simulink model "lab2_1"  (R2023b)
settings: Solver=VariableStepAuto  StartTime=0.0  StopTime=20.0  MaxStep=0.001  RelTol=1e-3
settings Model: Creator=insomnia  LastModifiedBy=insomnia

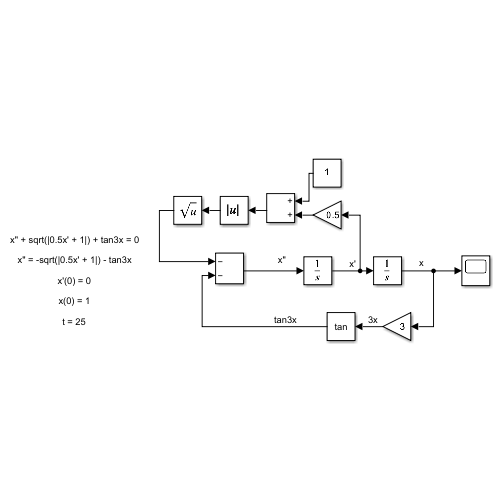
[thumbnail: Simulink's stored preview of the top-level diagram]
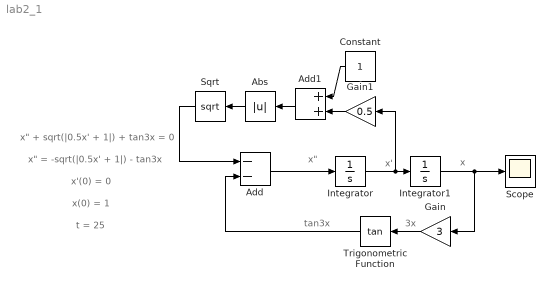
== system lab2_1 ==
  note: 3x
  note: tan3x
  note: x" + sqrt(|0.5x' + 1|) + tan3x = 0
  note: x" = -sqrt(|0.5x' + 1|) - tan3x
  note: x'
  note: x"
  note: x
  note: x'(0) = 0
  note: x(0) = 1
  note: t = 25
  Abs : Abs  SaturateOnIntegerOverflow=off
  Add : Sum  Inputs=--
  Add1 : Sum
  Constant : Constant
  Gain : Gain  Gain=3
  Gain1 : Gain  Gain=0.5
  Integrator : Integrator
  Integrator1 : Integrator  InitialCondition=1
  Scope : Scope
  Sqrt : Sqrt
  Trigonometric Function : Trigonometry  Operator=tan
  wires:
  Gain/1 -> Trigonometric Function/1
  Trigonometric Function/1 -> Add/2
  Sqrt/1 -> Add/1
  Abs/1 -> Sqrt/1
  Add/1 -> Integrator/1
  Integrator1/1 -> Gain/1, Scope/1
  Constant/1 -> Add1/1
  Integrator/1 -> Gain1/1, Integrator1/1
  Gain1/1 -> Add1/2
  Add1/1 -> Abs/1
